simulink model "Gesha1sluntukword"  (R2022b)
settings: Solver=VariableStepAuto  StartTime=0.0  StopTime=inf  RelTol=1e-3
undefined symbols (not defined in the file or in its folder): DiscIntNeverNeededParam
libraries: simulink x15, rllib x1
settings Model: Creator=yonat  LastModifiedBy=autom

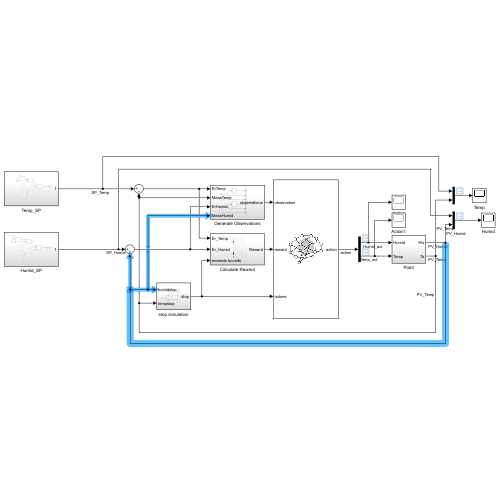
[thumbnail: Simulink's stored preview of the top-level diagram]
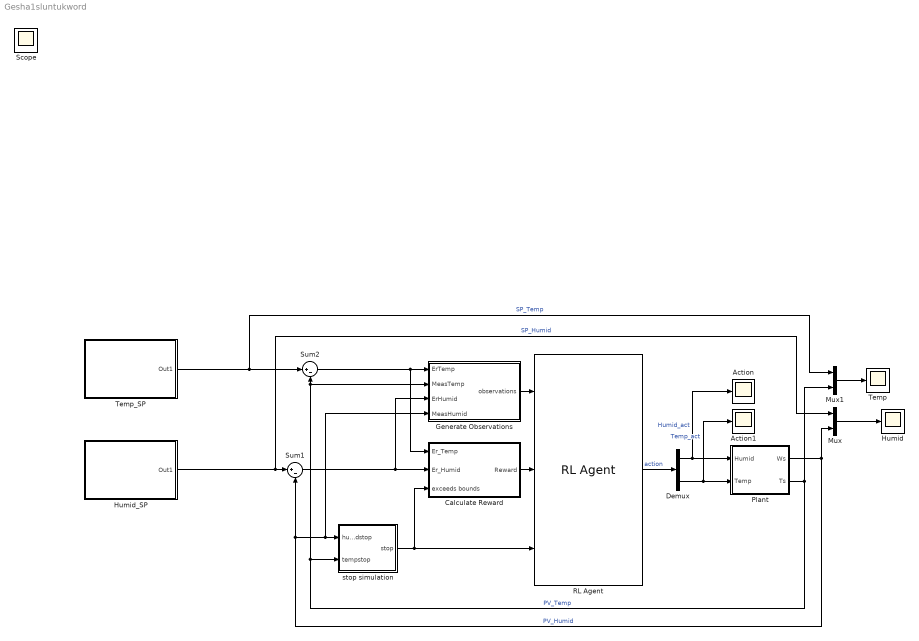
== system Gesha1sluntukword ==
  Action : Scope
  Action1 : Scope
  Calculate Reward : Subsystem
  Demux : Demux  Outputs=2
  Generate Observations : Subsystem
  Humid : Scope
  Humid_SP : Subsystem
  Mux : Mux  Inputs=2
  Mux1 : Mux  Inputs=2
  Plant : Subsystem
  RL Agent : rllib/RL Agent  Agent=agent  ExternalActionAsInput=off  ProvideLastAction=off  ProvideCumRwd=off  TreatAsDirectFeedthrough=on  UseStrictObservationDataTypes=off
  Sum1 : Sum  Inputs=|+-  SaturateOnIntegerOverflow=on
  Sum2 : Sum  Inputs=|+-  SaturateOnIntegerOverflow=on
  Temp : Scope
  Temp_SP : Subsystem
  stop simulation : Subsystem
  Scope : Scope
  wires:
  stop simulation/1(stop) -> Calculate Reward/3(exceeds bounds), RL Agent/3
  Plant/2(Ts) -> Mux1/2, Sum2/2, Generate Observations/2(MeasTemp), stop simulation/2(tempstop)  "PV_Temp"
  Sum2/1 -> Calculate Reward/1(Er_Temp), Generate Observations/1(ErTemp)
  Plant/1(Ws) -> Mux/2, Sum1/2, Generate Observations/4(MeasHumid), stop simulation/1(humidstop)  "PV_Humid"
  Sum1/1 -> Generate Observations/3(ErHumid), Calculate Reward/2(Er_Humid)
  RL Agent/1 -> Demux/1  "action"
  Generate Observations/1(observations) -> RL Agent/1
  Demux/2 -> Plant/2(Temp), Action1/1  "Temp_act"
  Demux/1 -> Action/1, Plant/1(Humid)  "Humid_act"
  Calculate Reward/1(Reward) -> RL Agent/2
  Mux/1 -> Humid/1
  Mux1/1 -> Temp/1
  Humid_SP/1(Out1) -> Mux/1, Sum1/1  "SP_Humid"
  Temp_SP/1(Out1) -> Mux1/1, Sum2/1  "SP_Temp"

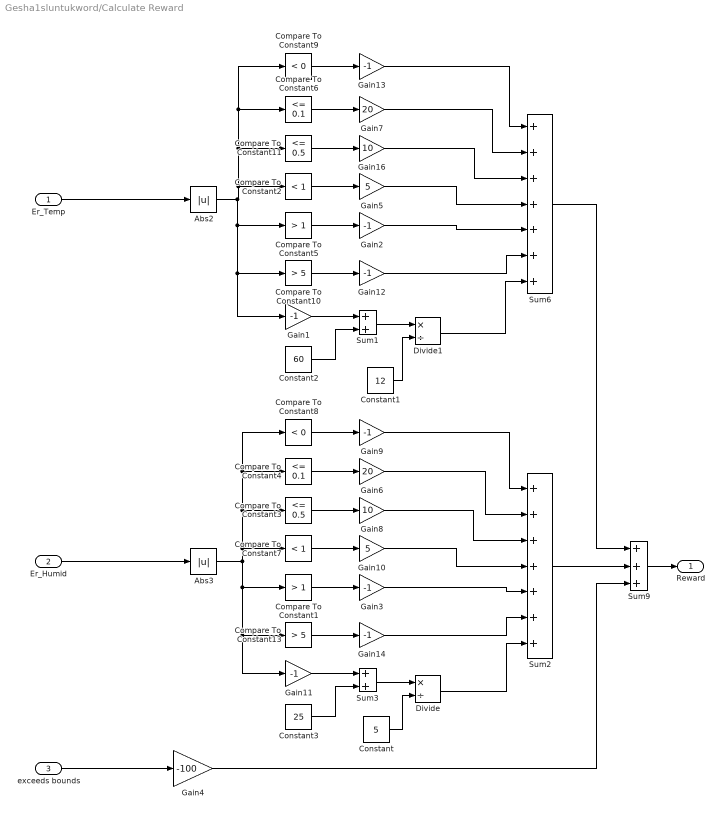
== system Gesha1sluntukword/Calculate Reward ==
  Er_Temp : Inport
  Er_Humid : Inport  Port=2
  exceeds bounds : Inport  Port=3
  Abs2 : Abs  SaturateOnIntegerOverflow=off
  Abs3 : Abs  SaturateOnIntegerOverflow=off
  Compare To Constant1 : simulink/Logic and Bit Operations/Compare To Constant  relop=>  const=1  OutDataTypeStr=boolean
  Compare To Constant10 : simulink/Logic and Bit Operations/Compare To Constant  relop=>  const=5  OutDataTypeStr=boolean
  Compare To Constant11 : simulink/Logic and Bit Operations/Compare To Constant  relop=<=  const=0.5  OutDataTypeStr=boolean
  Compare To Constant13 : simulink/Logic and Bit Operations/Compare To Constant  relop=>  const=5  OutDataTypeStr=boolean
  Compare To Constant2 : simulink/Logic and Bit Operations/Compare To Constant  relop=<  const=1  OutDataTypeStr=boolean
  Compare To Constant3 : simulink/Logic and Bit Operations/Compare To Constant  relop=<=  const=0.5  OutDataTypeStr=boolean
  Compare To Constant4 : simulink/Logic and Bit Operations/Compare To Constant  relop=<=  const=0.1  OutDataTypeStr=boolean
  Compare To Constant5 : simulink/Logic and Bit Operations/Compare To Constant  relop=>  const=1  OutDataTypeStr=boolean
  Compare To Constant6 : simulink/Logic and Bit Operations/Compare To Constant  relop=<=  const=0.1  OutDataTypeStr=boolean
  Compare To Constant7 : simulink/Logic and Bit Operations/Compare To Constant  relop=<  const=1  OutDataTypeStr=boolean
  Compare To Constant8 : simulink/Logic and Bit Operations/Compare To Constant  relop=<  const=0  OutDataTypeStr=boolean
  Compare To Constant9 : simulink/Logic and Bit Operations/Compare To Constant  relop=<  const=0  OutDataTypeStr=boolean
  Constant : Constant  Value=5
  Constant1 : Constant  Value=12
  Constant2 : Constant  Value=60
  Constant3 : Constant  Value=25
  Divide : Product  Inputs=*/
  Divide1 : Product  Inputs=*/
  Gain{1..3,9,11..14} (8 alike) : Gain  Gain=-1
  Gain10 : Gain  Gain=5
  Gain16 : Gain  Gain=10
  Gain4 : Gain  Gain=-100
  Gain5 : Gain  Gain=5
  Gain6 : Gain  Gain=20
  Gain7 : Gain  Gain=20
  Gain8 : Gain  Gain=10
  Sum1 : Sum
  Sum2 : Sum  Inputs=7
  Sum3 : Sum
  Sum6 : Sum  Inputs=7
  Sum9 : Sum  Inputs=+++
  Reward : Outport
  wires:
  Sum2/1 -> Sum9/2
  Er_Temp/1 -> Abs2/1
  Compare To Constant2/1 -> Gain5/1
  Compare To Constant13/1 -> Gain14/1
  Gain2/1 -> Sum6/5
  Sum9/1 -> Reward/1
  Gain8/1 -> Sum2/3
  Gain12/1 -> Sum6/6
  Compare To Constant11/1 -> Gain16/1
  Compare To Constant3/1 -> Gain8/1
  Er_Humid/1 -> Abs3/1
  Gain4/1 -> Sum9/3
  exceeds bounds/1 -> Gain4/1
  Compare To Constant10/1 -> Gain12/1
  Gain14/1 -> Sum2/6
  Gain10/1 -> Sum2/4
  Sum6/1 -> Sum9/1
  Gain16/1 -> Sum6/3
  Gain5/1 -> Sum6/4
  Gain11/1 -> Sum3/1
  Constant3/1 -> Sum3/2
  Constant/1 -> Divide/2
  Sum3/1 -> Divide/1
  Divide/1 -> Sum2/7
  Constant2/1 -> Sum1/2
  Sum1/1 -> Divide1/1
  Constant1/1 -> Divide1/2
  Gain1/1 -> Sum1/1
  Divide1/1 -> Sum6/7
  Compare To Constant1/1 -> Gain3/1
  Compare To Constant7/1 -> Gain10/1
  Gain3/1 -> Sum2/5
  Compare To Constant5/1 -> Gain2/1
  Compare To Constant4/1 -> Gain6/1
  Gain6/1 -> Sum2/2
  Gain7/1 -> Sum6/2
  Compare To Constant6/1 -> Gain7/1
  Abs3/1 -> Compare To Constant1/1, Gain11/1, Compare To Constant13/1, Compare To Constant8/1, Compare To Constant4/1, Compare To Constant3/1, Compare To Constant7/1
  Compare To Constant8/1 -> Gain9/1
  Gain9/1 -> Sum2/1
  Gain13/1 -> Sum6/1
  Compare To Constant9/1 -> Gain13/1
  Abs2/1 -> Compare To Constant5/1, Compare To Constant10/1, Gain1/1, Compare To Constant2/1, Compare To Constant9/1, Compare To Constant6/1, Compare To Constant11/1

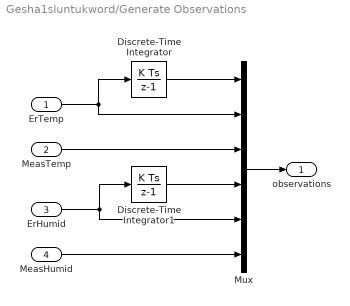
== system Gesha1sluntukword/Generate Observations ==
  ErTemp : Inport
  MeasTemp : Inport  Port=2
  ErHumid : Inport  Port=3
  MeasHumid : Inport  Port=4
  Discrete-Time Integrator : DiscreteIntegrator  SampleTime=1.0  ICPrevOutput=DiscIntNeverNeededParam  ICPrevScaledInput=DiscIntNeverNeededParam
  Discrete-Time Integrator1 : DiscreteIntegrator  SampleTime=1.0  ICPrevOutput=DiscIntNeverNeededParam  ICPrevScaledInput=DiscIntNeverNeededParam
  Mux : Mux  Inputs=6
  observations : Outport  VectorParamsAs1DForOutWhenUnconnected=off
  wires:
  ErTemp/1 -> Discrete-Time Integrator/1, Mux/2
  ErHumid/1 -> Mux/5, Discrete-Time Integrator1/1
  Discrete-Time Integrator1/1 -> Mux/4
  Discrete-Time Integrator/1 -> Mux/1
  MeasTemp/1 -> Mux/3
  MeasHumid/1 -> Mux/6
  Mux/1 -> observations/1

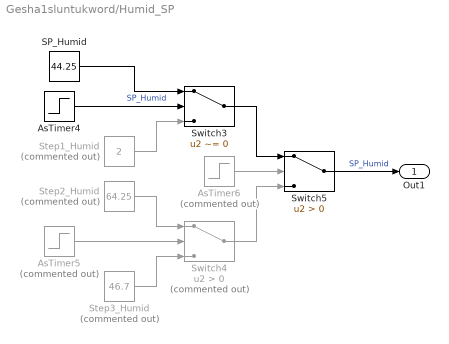
== system Gesha1sluntukword/Humid_SP ==
  AsTimer4 : Step  Time=5000  Before=1  After=0  SampleTime=0
  AsTimer5 : Step  Commented=on  Time=600  Before=1  After=0  SampleTime=0
  AsTimer6 : Step  Commented=on  Time=5000  Before=1  After=0  SampleTime=0
  SP_Humid : Constant  Value=44.25
  Step1_Humid : Constant  Commented=on  Value=2
  Step2_Humid : Constant  Commented=on  Value=64.25
  Step3_Humid : Constant  Commented=on  Value=46.7
  Switch3 : Switch  Criteria=u2 ~= 0  Threshold=1  SaturateOnIntegerOverflow=off  InputSameDT=off
  Switch4 : Switch  Commented=on  Criteria=u2 > Threshold  SaturateOnIntegerOverflow=off  InputSameDT=off
  Switch5 : Switch  Criteria=u2 > Threshold  SaturateOnIntegerOverflow=off  InputSameDT=off
  Out1 : Outport
  wires:
  SP_Humid/1 -> Switch3/1  "SP_Humid"
  Step1_Humid/1 -> Switch3/3
  Step2_Humid/1 -> Switch4/1
  Switch3/1 -> Switch5/1
  Step3_Humid/1 -> Switch4/3
  AsTimer6/1 -> Switch5/2
  Switch4/1 -> Switch5/3
  AsTimer4/1 -> Switch3/2
  AsTimer5/1 -> Switch4/2
  Switch5/1 -> Out1/1  "SP_Humid"

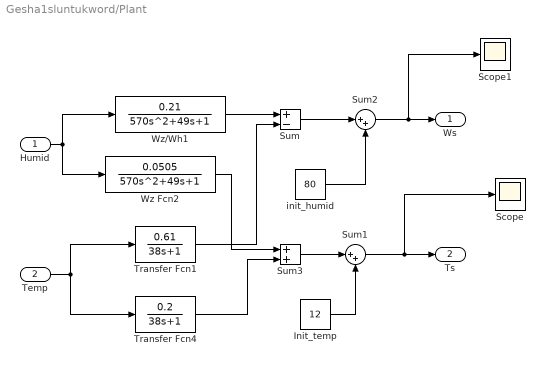
== system Gesha1sluntukword/Plant ==
  Humid : Inport
  Temp : Inport  Port=2
  Init_temp : Constant  Value=12
  Scope : Scope
  Scope1 : Scope
  Sum : Sum  Inputs=+-
  Sum1 : Sum  Inputs=|++
  Sum2 : Sum  Inputs=|++
  Sum3 : Sum
  Transfer Fcn1 : TransferFcn  Numerator=[0.61]  Denominator=[38 1]
  Transfer Fcn4 : TransferFcn  Numerator=[0.2]  Denominator=[38 1]
  Wz Fcn2 : TransferFcn  Numerator=[0.0505]  Denominator=[570 49 1]
  Wz/Wh1 : TransferFcn  Numerator=[0.21]  Denominator=[570 49 1]
  init_humid : Constant  Value=80
  Ws : Outport
  Ts : Outport  Port=2
  wires:
  Wz Fcn2/1 -> Sum3/1
  Humid/1 -> Wz/Wh1/1, Wz Fcn2/1
  Temp/1 -> Transfer Fcn1/1, Transfer Fcn4/1
  Transfer Fcn1/1 -> Sum/2
  Wz/Wh1/1 -> Sum/1
  Transfer Fcn4/1 -> Sum3/2
  Sum/1 -> Sum2/1
  Sum3/1 -> Sum1/1
  Sum1/1 -> Scope/1, Ts/1
  Sum2/1 -> Scope1/1, Ws/1
  Init_temp/1 -> Sum1/2
  init_humid/1 -> Sum2/2

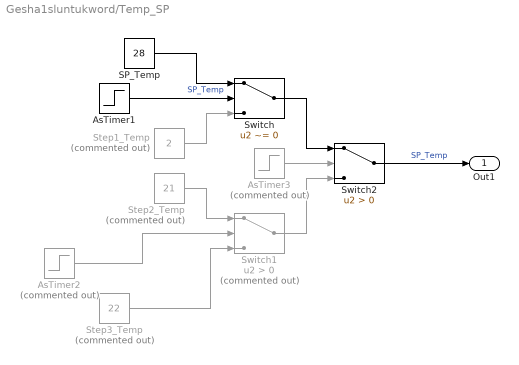
== system Gesha1sluntukword/Temp_SP ==
  AsTimer1 : Step  Time=5000  Before=1  After=0  SampleTime=0
  AsTimer2 : Step  Commented=on  Time=600  Before=1  After=0  SampleTime=0
  AsTimer3 : Step  Commented=on  Time=5000  Before=1  After=0  SampleTime=0
  SP_Temp : Constant  Value=28
  Step1_Temp : Constant  Commented=on  Value=2
  Step2_Temp : Constant  Commented=on  Value=21
  Step3_Temp : Constant  Commented=on  Value=22
  Switch : Switch  Criteria=u2 ~= 0  Threshold=1  SaturateOnIntegerOverflow=off  InputSameDT=off
  Switch1 : Switch  Commented=on  Criteria=u2 > Threshold  SaturateOnIntegerOverflow=off  InputSameDT=off
  Switch2 : Switch  Criteria=u2 > Threshold  SaturateOnIntegerOverflow=off  InputSameDT=off
  Out1 : Outport
  wires:
  SP_Temp/1 -> Switch/1  "SP_Temp"
  Switch/1 -> Switch2/1
  AsTimer1/1 -> Switch/2
  Step2_Temp/1 -> Switch1/1
  AsTimer2/1 -> Switch1/2
  AsTimer3/1 -> Switch2/2
  Step1_Temp/1 -> Switch/3
  Switch1/1 -> Switch2/3
  Step3_Temp/1 -> Switch1/3
  Switch2/1 -> Out1/1  "SP_Temp"

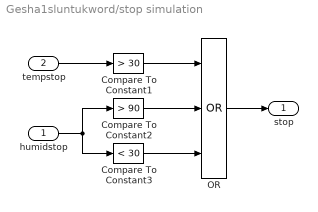
== system Gesha1sluntukword/stop simulation ==
  humidstop : Inport
  tempstop : Inport  Port=2
  Compare To Constant1 : simulink/Logic and Bit Operations/Compare To Constant  relop=>  const=30  OutDataTypeStr=boolean
  Compare To Constant2 : simulink/Logic and Bit Operations/Compare To Constant  relop=>  const=90  OutDataTypeStr=boolean
  Compare To Constant3 : simulink/Logic and Bit Operations/Compare To Constant  relop=<  const=30  OutDataTypeStr=boolean
  OR : Logic  Operator=OR  Inputs=3  IconShape=distinctive  AllPortsSameDT=off  OutDataTypeStr=boolean
  stop : Outport  VectorParamsAs1DForOutWhenUnconnected=off
  wires:
  tempstop/1 -> Compare To Constant1/1
  humidstop/1 -> Compare To Constant2/1, Compare To Constant3/1
  Compare To Constant1/1 -> OR/1
  Compare To Constant3/1 -> OR/3
  OR/1 -> stop/1
  Compare To Constant2/1 -> OR/2
